simulink model "tv_system_sq2_4"  (R2021b)
settings: Solver=VariableStepAuto  StartTime=0.0  StopTime=0  RelTol=1e-3
values from neighbouring files (symbols this model uses):
  gamma1 = 0.005    [main_pixloss.m]
  gamma2 = 1/(1.05*tau2)*(1/gamma1-beta/2)    [main_pixloss.m]
  lambda = 0.012    [main_pixloss.m]
  maxIter = 500    [main_pixloss.m]
undefined symbols (not defined in the file or in its folder): cols, rows
libraries: visionsources x3, visionstatistics x2
settings Model: Creator=abeshu  LastModifiedBy=shu_abe

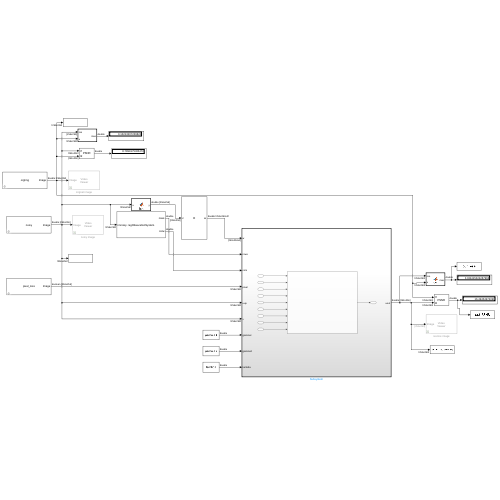
[thumbnail: Simulink's stored preview of the top-level diagram]
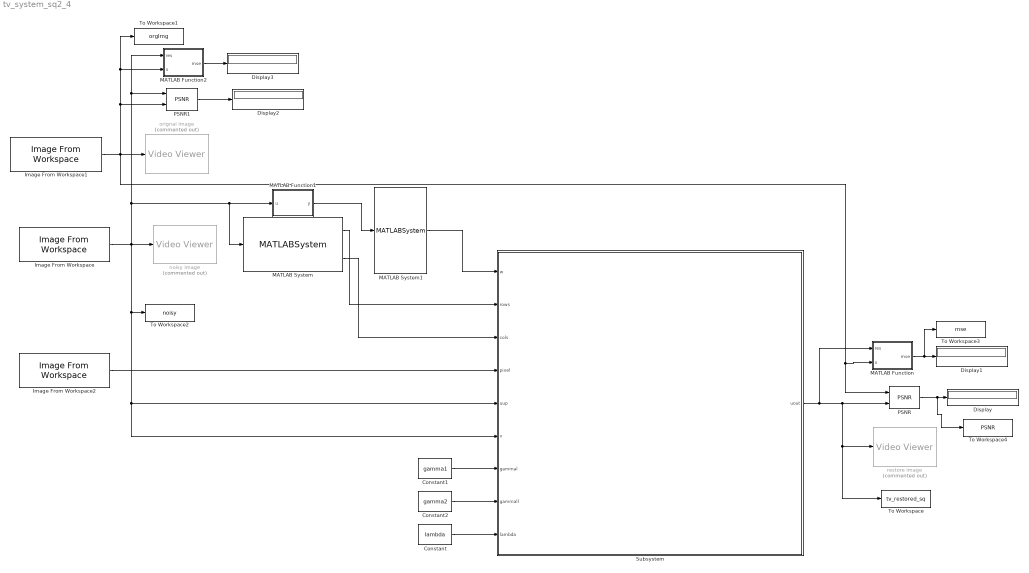
== system tv_system_sq2_4 ==
  Constant : Constant  Value=lambda
  Constant1 : Constant  Value=gamma1
  Constant2 : Constant  Value=gamma2
  Display{,1..3} (4 alike) : Display
  Image From Workspace : visionsources/Image From Workspace  Tag=vipblks_nd  ImageValue=noisy  Ts=inf  imagePorts=One multidimensional signal  OutPortLabels=R|G|B  ImageDataType=Inherit from 'Value'  Signed=on  WordLength=16  sdImageDataType=sfix(16)  FractionLengthMode=User-defined  FractionLength=15
      settings: SourceProductBaseCode=VP
  Image From Workspace1 : visionsources/Image From Workspace  Tag=vipblks_nd  ImageValue=orgImg  Ts=inf  imagePorts=One multidimensional signal  OutPortLabels=R|G|B  ImageDataType=Inherit from 'Value'  Signed=on  WordLength=16  sdImageDataType=sfix(16)  FractionLengthMode=User-defined  FractionLength=15
      settings: SourceProductBaseCode=VP
  Image From Workspace2 : visionsources/Image From Workspace  Tag=vipblks_nd  ImageValue=pixel_loss  Ts=inf  imagePorts=One multidimensional signal  OutPortLabels=R|G|B  ImageDataType=Inherit from 'Value'  Signed=on  WordLength=16  sdImageDataType=sfix(16)  FractionLengthMode=User-defined  FractionLength=15
      settings: SourceProductBaseCode=VP
  MATLAB Function : MATLAB Function  TreatAsAtomicUnit=on
  MATLAB Function1 : MATLAB Function  TreatAsAtomicUnit=on
  MATLAB Function2 : MATLAB Function  TreatAsAtomicUnit=on
  MATLAB System : MATLABSystem  System=regObsevationSystem  SimulateUsing=Code generation
      mask Type: regObsevationSystem
      mask Display:
      | disp('regObsevationSystem');
      | port_label('input',1,'imnoisy');
      | port_label('output',1,'rows');
      | port_label('output',2,'colw');
  MATLAB System1 : MATLABSystem  System=dBlockSystem  SimulateUsing=Code generation
      mask Type: dBlockSystem
      mask Display:
      | disp('D');
      | port_label('input',1,'z');
      | port_label('output',1,'w');
  PSNR : visionstatistics/PSNR
      settings: SourceProductBaseCode=VP
  PSNR1 : visionstatistics/PSNR
      settings: SourceProductBaseCode=VP
  Subsystem : Subsystem  TreatAsAtomicUnit=on
  To Workspace : ToWorkspace  VariableName=tv_restored_sq  SaveFormat=Structure  SampleTime=-1
      settings: Save2DSignal=2-D array (concatenate along first dimension)
  To Workspace1 : ToWorkspace  VariableName=orgImg  SaveFormat=Structure  SampleTime=-1
      settings: Save2DSignal=2-D array (concatenate along first dimension)
  To Workspace2 : ToWorkspace  VariableName=noisy  SaveFormat=Structure  SampleTime=-1
      settings: Save2DSignal=2-D array (concatenate along first dimension)
  To Workspace3 : ToWorkspace  VariableName=mse  SaveFormat=Structure  SampleTime=-1
      settings: Save2DSignal=2-D array (concatenate along first dimension)
  To Workspace4 : ToWorkspace  VariableName=PSNR  SaveFormat=Structure  SampleTime=-1
      settings: Save2DSignal=2-D array (concatenate along first dimension)
  noisy image : VideoViewer  Commented=on  FigPos=[349 1002 318 374]
  orignal image : VideoViewer  Commented=on  FigPos=[263 689 480 338]
  restore image : VideoViewer  Commented=on  FigPos=[325 861 538 407]
  wires:
  Image From Workspace/1 -> To Workspace2/1, Subsystem/6(v), Subsystem/5(uup), MATLAB Function2/1(res), PSNR1/1, MATLAB System/1, MATLAB Function1/1(u), noisy image/1
  Image From Workspace1/1 -> To Workspace1/1, MATLAB Function2/2(u), PSNR1/2, MATLAB Function/2(u), PSNR/1, orignal image/1
  Image From Workspace2/1 -> Subsystem/4(pixel)
  MATLAB System/1 -> Subsystem/2(rows)
  MATLAB System/2 -> Subsystem/3(cols)
  MATLAB Function1/1(y) -> MATLAB System1/1
  Constant1/1 -> Subsystem/7(gammal)
  Constant2/1 -> Subsystem/8(gammall)
  Constant/1 -> Subsystem/9(lambda)
  MATLAB System1/1 -> Subsystem/1(w)
  Subsystem/1(uout) -> To Workspace/1, restore image/1, PSNR/2, MATLAB Function/1(res)
  PSNR/1 -> To Workspace4/1, Display/1
  MATLAB Function/1(mse) -> To Workspace3/1, Display1/1
  PSNR1/1 -> Display2/1
  MATLAB Function2/1(mse) -> Display3/1

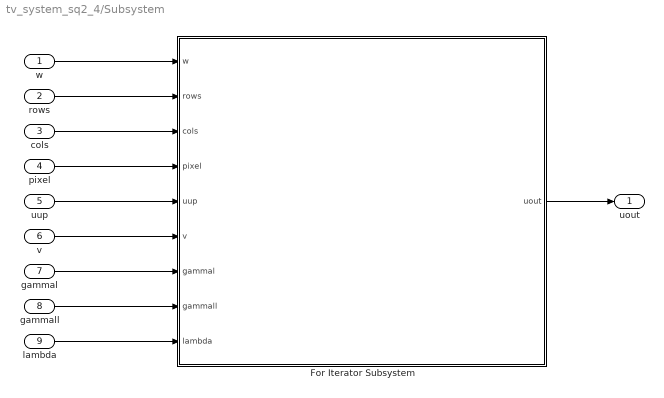
== system tv_system_sq2_4/Subsystem ==
  w : Inport
  rows : Inport  Port=2
  cols : Inport  Port=3
  pixel : Inport  Port=4
  uup : Inport  Port=5
  v : Inport  Port=6
  gammal : Inport  Port=7
  gammall : Inport  Port=8
  lambda : Inport  Port=9
  For Iterator Subsystem : Subsystem  TreatAsAtomicUnit=on
  uout : Outport
  wires:
  For Iterator Subsystem/1(uout) -> uout/1
  w/1 -> For Iterator Subsystem/1(w)
  rows/1 -> For Iterator Subsystem/2(rows)
  cols/1 -> For Iterator Subsystem/3(cols)
  pixel/1 -> For Iterator Subsystem/4(pixel)
  uup/1 -> For Iterator Subsystem/5(uup)
  v/1 -> For Iterator Subsystem/6(v)
  gammal/1 -> For Iterator Subsystem/7(gammal)
  gammall/1 -> For Iterator Subsystem/8(gammall)
  lambda/1 -> For Iterator Subsystem/9(lambda)

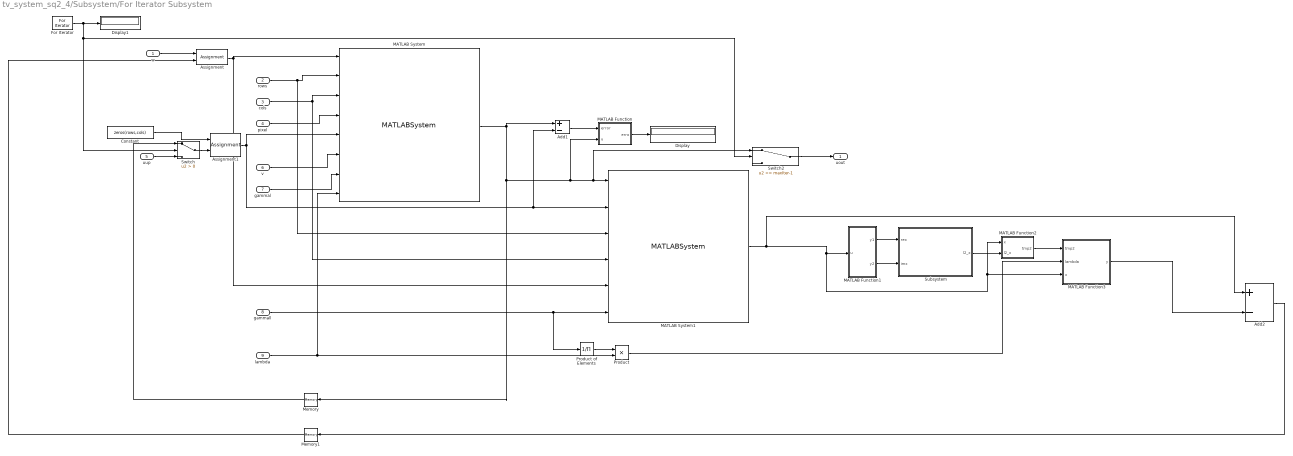
== system tv_system_sq2_4/Subsystem/For Iterator Subsystem ==
  w : Inport
  rows : Inport  Port=2
  cols : Inport  Port=3
  pixel : Inport  Port=4
  uup : Inport  Port=5
  v : Inport  Port=6
  gammal : Inport  Port=7
  gammall : Inport  Port=8
  lambda : Inport  Port=9
  Add1 : Sum  Inputs=+-
  Add2 : Sum  Inputs=+-
  Assignment : Assignment  NumberOfDimensions=3  DiagnosticForDimensions=Warning  IndexOptions=Assign all,Assign all,Assign all  Indices=1,1,1  OutputSizes=1,1,1
  Assignment1 : Assignment  NumberOfDimensions=2  DiagnosticForDimensions=Warning  IndexOptions=Assign all,Assign all  Indices=1,1  OutputSizes=1,1
  Constant : Constant  Value=zeros(rows,cols)
  Display : Display
  Display1 : Display
  For Iterator : ForIterator  IterationLimit=maxIter  IndexMode=Zero-based  IterationVariableDataType=double
  MATLAB Function : MATLAB Function  TreatAsAtomicUnit=on
  MATLAB Function1 : MATLAB Function  TreatAsAtomicUnit=on
  MATLAB Function2 : MATLAB Function  TreatAsAtomicUnit=on
  MATLAB Function3 : MATLAB Function  TreatAsAtomicUnit=on
  MATLAB System : MATLABSystem  System=updateuSystem  SimulateUsing=Code generation
      mask Type: updateuSystem
      mask Display:
      | disp('updateuSystem');
      | port_label('input',1,'w');
      | port_label('input',2,'rows');
      | port_label('input',3,'cols');
      | port_label('input',4,'pixel');
      | port_label('input',5,'uup');
      | port_label('input',6,'v');
      | port_label('input',7,'gamma1');
      | port_label('input',8,'lambda');
      | port_label('output',1,'u');
  MATLAB System1 : MATLABSystem  System=updatewSystem  SimulateUsing=Code generation
      mask Type: updatewSystem
      mask Display:
      | disp('updatewSystem');
      | port_label('input',1,'u');
      | port_label('input',2,'upre');
      | port_label('input',3,'rows');
      | port_label('input',4,'cols');
      | port_label('input',5,'w');
      | port_label('input',6,'gamma2');
      | port_label('output',1,'w_tilde');
  Memory : Memory  InheritSampleTime=on
  Memory1 : Memory  InheritSampleTime=on
  Product : Product
  Product of Elements : Product  Inputs=/
  Subsystem : Subsystem
  Switch : Switch  Criteria=u2 > Threshold
  Switch2 : Switch  Threshold=maxIter-1
  uout : Outport
  wires:
  w/1 -> Assignment/1
  Assignment/1 -> MATLAB System/1, MATLAB System1/5
  rows/1 -> MATLAB System/2, MATLAB System1/3
  cols/1 -> MATLAB System1/4, MATLAB System/3
  pixel/1 -> MATLAB System/4
  Constant/1 -> Assignment1/1
  Switch/1 -> Assignment1/2
  uup/1 -> Switch/3
  Assignment1/1 -> Add1/2, MATLAB System1/2, MATLAB System/5
  v/1 -> MATLAB System/6
  gammal/1 -> MATLAB System/7
  For Iterator/1 -> Switch/2, Switch2/2, Display1/1
  MATLAB System/1 -> Add1/1, Switch2/1, MATLAB System1/1, MATLAB Function/2(u), Memory/1
  Add1/1 -> MATLAB Function/1(error)
  MATLAB Function/1(erro) -> Display/1
  gammall/1 -> Product of Elements/1, MATLAB System1/6
  MATLAB Function1/1(y1) -> Subsystem/1(rex)
  MATLAB System1/1 -> MATLAB Function3/3(x), MATLAB Function2/1(x), MATLAB Function1/1(u), Add2/1
  Subsystem/1(l2_x) -> MATLAB Function2/2(l2_x)
  MATLAB Function2/1(tmp2) -> MATLAB Function3/1(tmp2)
  Product of Elements/1 -> Product/1
  lambda/1 -> MATLAB System/8, Product/2
  Product/1 -> MATLAB Function3/2(lambda)
  Memory/1 -> Switch/1
  Add2/1 -> Memory1/1
  MATLAB Function3/1(y) -> Add2/2
  Memory1/1 -> Assignment/2
  Switch2/1 -> uout/1
  MATLAB Function1/2(y2) -> Subsystem/2(imx)

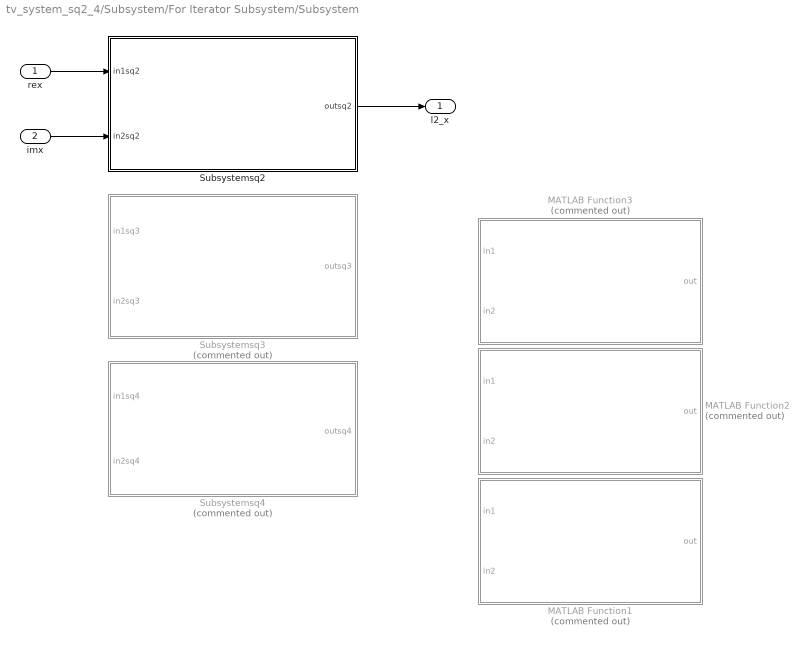
== system tv_system_sq2_4/Subsystem/For Iterator Subsystem/Subsystem ==
  rex : Inport
  imx : Inport  Port=2
  MATLAB Function1 : MATLAB Function  Commented=on  TreatAsAtomicUnit=on
  MATLAB Function2 : MATLAB Function  Commented=on  TreatAsAtomicUnit=on
  MATLAB Function3 : MATLAB Function  Commented=on  TreatAsAtomicUnit=on
  Subsystemsq2 : Subsystem
  Subsystemsq3 : Subsystem  Commented=on
  Subsystemsq4 : Subsystem  Commented=on
  l2_x : Outport
  wires:
  rex/1 -> Subsystemsq2/1(in1sq2)
  imx/1 -> Subsystemsq2/2(in2sq2)
  Subsystemsq2/1(outsq2) -> l2_x/1

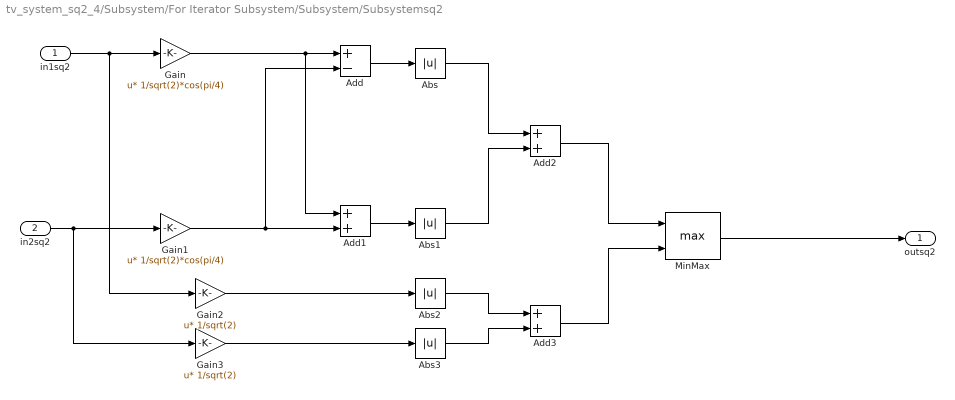
== system tv_system_sq2_4/Subsystem/For Iterator Subsystem/Subsystem/Subsystemsq2 ==
  in1sq2 : Inport
  in2sq2 : Inport  Port=2
  Abs{,1..3} (4 alike) : Abs
  Add : Sum  Inputs=+-
  Add1 : Sum
  Add2 : Sum
  Add3 : Sum
  Gain : Gain  Gain=1/sqrt(2)*cos(pi/4)  Multiplication=Matrix(u*K)
  Gain1 : Gain  Gain=1/sqrt(2)*cos(pi/4)  Multiplication=Matrix(u*K)
  Gain2 : Gain  Gain=1/sqrt(2)  Multiplication=Matrix(u*K)
  Gain3 : Gain  Gain=1/sqrt(2)  Multiplication=Matrix(u*K)
  MinMax : MinMax  Function=max  Inputs=2
  outsq2 : Outport
  wires:
  Gain/1 -> Add1/1, Add/1
  Add/1 -> Abs/1
  MinMax/1 -> outsq2/1
  Add3/1 -> MinMax/2
  Abs1/1 -> Add2/2
  Add2/1 -> MinMax/1
  Abs/1 -> Add2/1
  in1sq2/1 -> Gain2/1, Gain/1
  Gain1/1 -> Add1/2, Add/2
  in2sq2/1 -> Gain3/1, Gain1/1
  Abs3/1 -> Add3/2
  Add1/1 -> Abs1/1
  Abs2/1 -> Add3/1
  Gain2/1 -> Abs2/1
  Gain3/1 -> Abs3/1

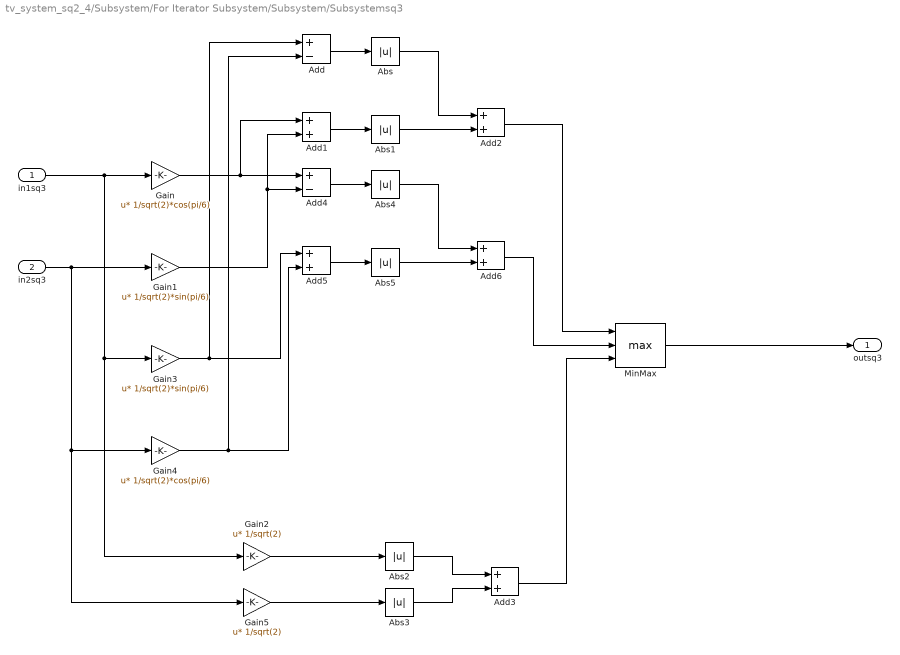
== system tv_system_sq2_4/Subsystem/For Iterator Subsystem/Subsystem/Subsystemsq3 ==
  in1sq3 : Inport
  in2sq3 : Inport  Port=2
  Abs{,1..5} (6 alike) : Abs
  Add : Sum  Inputs=+-
  Add{1..3,5..6} (5 alike) : Sum
  Add4 : Sum  Inputs=+-
  Gain : Gain  Gain=1/sqrt(2)*cos(pi/6)  Multiplication=Matrix(u*K)
  Gain1 : Gain  Gain=1/sqrt(2)*sin(pi/6)  Multiplication=Matrix(u*K)
  Gain2 : Gain  Gain=1/sqrt(2)  Multiplication=Matrix(u*K)
  Gain3 : Gain  Gain=1/sqrt(2)*sin(pi/6)  Multiplication=Matrix(u*K)
  Gain4 : Gain  Gain=1/sqrt(2)*cos(pi/6)  Multiplication=Matrix(u*K)
  Gain5 : Gain  Gain=1/sqrt(2)  Multiplication=Matrix(u*K)
  MinMax : MinMax  Function=max  Inputs=3
  outsq3 : Outport
  wires:
  MinMax/1 -> outsq3/1
  Abs/1 -> Add2/1
  Abs1/1 -> Add2/2
  Abs4/1 -> Add6/1
  Add4/1 -> Abs4/1
  Gain/1 -> Add4/1, Add1/1
  in2sq3/1 -> Gain5/1, Gain4/1, Gain1/1
  Gain4/1 -> Add/2, Add5/2
  Abs3/1 -> Add3/2
  Gain3/1 -> Add/1, Add5/1
  Add6/1 -> MinMax/2
  Gain1/1 -> Add4/2, Add1/2
  in1sq3/1 -> Gain3/1, Gain2/1, Gain/1
  Abs5/1 -> Add6/2
  Add1/1 -> Abs1/1
  Add3/1 -> MinMax/3
  Abs2/1 -> Add3/1
  Add/1 -> Abs/1
  Add5/1 -> Abs5/1
  Add2/1 -> MinMax/1
  Gain2/1 -> Abs2/1
  Gain5/1 -> Abs3/1

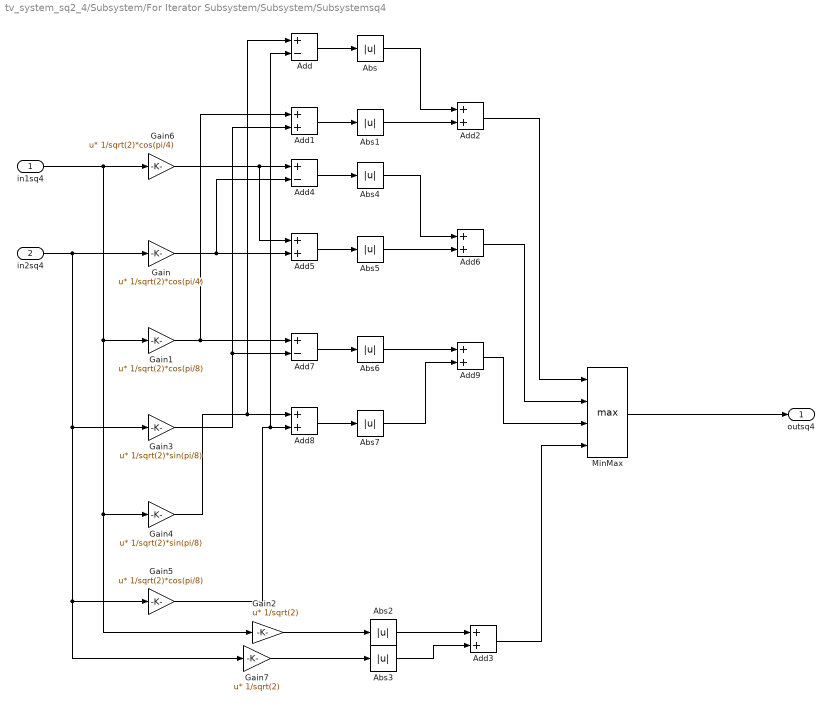
== system tv_system_sq2_4/Subsystem/For Iterator Subsystem/Subsystem/Subsystemsq4 ==
  in1sq4 : Inport
  in2sq4 : Inport  Port=2
  Abs{,1..7} (8 alike) : Abs
  Add : Sum  Inputs=+-
  Add{1..3,5..6,8..9} (7 alike) : Sum
  Add4 : Sum  Inputs=+-
  Add7 : Sum  Inputs=+-
  Gain : Gain  Gain=1/sqrt(2)*cos(pi/4)  Multiplication=Matrix(u*K)
  Gain1 : Gain  Gain=1/sqrt(2)*cos(pi/8)  Multiplication=Matrix(u*K)
  Gain2 : Gain  Gain=1/sqrt(2)  Multiplication=Matrix(u*K)
  Gain3 : Gain  Gain=1/sqrt(2)*sin(pi/8)  Multiplication=Matrix(u*K)
  Gain4 : Gain  Gain=1/sqrt(2)*sin(pi/8)  Multiplication=Matrix(u*K)
  Gain5 : Gain  Gain=1/sqrt(2)*cos(pi/8)  Multiplication=Matrix(u*K)
  Gain6 : Gain  Gain=1/sqrt(2)*cos(pi/4)  Multiplication=Matrix(u*K)
  Gain7 : Gain  Gain=1/sqrt(2)  Multiplication=Matrix(u*K)
  MinMax : MinMax  Function=max  Inputs=4
  outsq4 : Outport
  wires:
  Abs/1 -> Add2/1
  Gain1/1 -> Add7/1, Add1/1
  Abs6/1 -> Add9/1
  Abs5/1 -> Add6/2
  Add6/1 -> MinMax/2
  Gain4/1 -> Add8/1, Add/1
  Gain3/1 -> Add1/2, Add7/2
  in2sq4/1 -> Gain5/1, Gain7/1, Gain3/1, Gain/1
  Gain/1 -> Add5/2, Add4/2
  Add5/1 -> Abs5/1
  in1sq4/1 -> Gain1/1, Gain2/1, Gain4/1, Gain6/1
  Add3/1 -> MinMax/4
  Add7/1 -> Abs6/1
  Add8/1 -> Abs7/1
  Add2/1 -> MinMax/1
  Add4/1 -> Abs4/1
  Gain5/1 -> Add8/2, Add/2
  Abs2/1 -> Add3/1
  Abs7/1 -> Add9/2
  Add1/1 -> Abs1/1
  Add9/1 -> MinMax/3
  Abs3/1 -> Add3/2
  Abs4/1 -> Add6/1
  MinMax/1 -> outsq4/1
  Add/1 -> Abs/1
  Gain6/1 -> Add4/1, Add5/1
  Abs1/1 -> Add2/2
  Gain2/1 -> Abs2/1
  Gain7/1 -> Abs3/1

== matlab function tv_system_sq2_4/Subsystem/For Iterator Subsystem/MATLAB Function2 ==
  data: x input; tmp2 output; l2_x input
function tmp2 = fcn(x,l2_x)

if isfi(x) == true
    tmp2 = divide(x.numerictype,1,l2_x);
else
    tmp2 = 1./l2_x;
end

== matlab function tv_system_sq2_4/Subsystem/For Iterator Subsystem/MATLAB Function ==
  data: error input; u input; erro output
function erro = fcn(error,u)

erro = norm(error(:),2) / norm(u(:),2);

== matlab function tv_system_sq2_4/Subsystem/For Iterator Subsystem/MATLAB Function3 ==
  data: tmp2 input; y output; lambda input; x input
function y = fcn(tmp2,lambda,x)

% tmp3 = lambda*tmp2;
y = repmat(max(1 - tmp2,0),1,1,2) .* x;

== matlab function tv_system_sq2_4/MATLAB Function ==
  data: res input; u input; mse output
function mse = fcn(res,u)

mse = immse(u,res);

== matlab function tv_system_sq2_4/Subsystem/For Iterator Subsystem/MATLAB Function1 ==
  data: u input; y1 output; y2 output
function [y1,y2] = fcn(u)
    y1 = u(:,:,1);
    y2 = u(:,:,2);
end

== matlab function tv_system_sq2_4/Subsystem/For Iterator Subsystem/Subsystem/MATLAB Function3 ==
  data: in1 input; out output; in2 input
function out = abssq04(in1,in2)

SIN_PI_4 = sin(pi/4);
COS_PI_4 = sin(pi/4);

% theta = 0
a0 = abs(in1) + abs(in2);
% theta = pi/4
a1 = abs(COS_PI_4*in1 - SIN_PI_4*in2) ...
    + abs(SIN_PI_4*in1 + COS_PI_4*in2);


out = (1/sqrt(2)).*max(a0, a1);

end

== matlab function tv_system_sq2_4/Subsystem/For Iterator Subsystem/Subsystem/MATLAB Function2 ==
  data: in1 input; out output; in2 input
function out = abssq06(in1,in2)

SIN_PI_6 = sin(pi/6);
SIN_2PI_6 = sin(2*pi/6);
COS_PI_6 = cos(pi/6);
COS_2PI_6 = cos(2*pi/6);

% Real and imaginary part


% theta = 0
a0 = abs(in1) + abs(in2);
% theta = pi/4
%a1 = abs(COS_PI_4*in1 - SIN_PI_4*in2) ...
%    + abs(SIN_PI_4*in1 + COS_PI_4*in2);

% theta = pi/6
a1 = abs(COS_PI_6*in1 - SIN_PI_6*in2) + abs(SIN_PI_6*in1 + COS_PI_6*in2);
% theta = 2pi/6
a2 = abs(COS_2PI_6*in1 - SIN_2PI_6*in2) + abs(SIN_2PI_6*in1 + COS_2PI_6*in2);


out = (1/sqrt(2)).*max(max(a0, a1),a2);

end

== matlab function tv_system_sq2_4/MATLAB Function2 ==
  data: res input; u input; mse output
function mse = fcn(res,u)

mse = immse(u,res);

== matlab function tv_system_sq2_4/Subsystem/For Iterator Subsystem/Subsystem/MATLAB Function1 ==
  data: in1 input; out output; in2 input
function out = abssq08(in1,in2)

SIN_PI_8 = sin(pi/8);
COS_PI_8 = cos(pi/8);

SIN_2PI_8 = sin(2*pi/8);
COS_2PI_8 = cos(2*pi/8);

SIN_3PI_8 = sin(3*pi/8);
COS_3PI_8 = cos(3*pi/8);

% Real and imaginary part

% theta = 0
a0 = abs(in1) + abs(in2);

% theta = pi/8
a1 = abs(COS_PI_8*in1 - SIN_PI_8*in2) + abs(SIN_PI_8*in1 + COS_PI_8*in2);
% theta = 2pi/8
a2 = abs(COS_2PI_8*in1 - SIN_2PI_8*in2) + abs(SIN_2PI_8*in1 + COS_2PI_8*in2);
% theta = 3pi/8
a3 = abs(COS_3PI_8*in1 - SIN_3PI_8*in2) + abs(SIN_3PI_8*in1 + COS_3PI_8*in2);


out = (1/sqrt(2)).*max(max(max(a0, a1),a2),a3);


end

== matlab function tv_system_sq2_4/MATLAB Function1 ==
  data: u input; y output
function y = fcn(u)

y = zeros(size(u));
